simulink model "RobotX_SLAMonly"  (R2014a)
settings: Solver=FixedStepDiscrete  StartTime=0.0  StopTime=inf  FixedStep=.25  RelTol=1e-3
undefined symbols (not defined in the file): Com1, Com2, Com3, Com4, DiscIntNeverNeededParam, standard
libraries: xpcseriallib x11, simulink x3, slrtlib x3, dspmtrx3 x2, speedgoatlib x1, speedgoatlib_IO102 x1
(part 8 of 15)

== matlab function RobotX_SLAMonly/Main FSM/SLAM/Models for prediction/Model46/Dynamic Model ==
  data: F_surge input; F_sway input; Torque input; u input; surgeAccel output; v input; psi input; swayAccel output; yawAccel output
function [surgeAccel, swayAccel, yawAccel] = ...
    WAM_V_3DOF(F_surge, F_sway, Torque, u, v, psi)
%Written by Anderson Lebbad on August 12, 2014
%Last Edited:

%This function was heavily based off of Ariel Qu's Vel3DOF_IvanV1. It was
%rewritten for real-time use.

%This function will produce the transient output surge velocity of a
%linearized model of the USV. It is assumed that the vehicle is equivalent
%to two cylinders in the water.

%%%%%DEFINED VARIABLE%%%%%%
%
%   Xext = Thrust from motors
%   Next = Moment from motor
%   m = Mass of vehicle
%   Xudot = Added mass in surge direction
%   Yvdot = Added mass in sway direction
%   Nrdot = Added mass from yaw
%   xg = offset from center of gravity
%   rho = density of seawater
%   S = wetted surface area
%   R = Reynolds number
%   Cd = Coefficient of drag
%   Cdc = Coefficient of drag for sway
%   nu = Kinematic viscosity
%   L = Length overall
%   T = draft
%   B = beam
%   SA = Surface area of cylinder experiencing sway
%   Iz = moment of inertia about Z axis
%
%%%%%%

% Force/Mometns from thrusters & control surfaces...

tau = [F_surge; F_sway; Torque];

% Calculate yaw rate
persistent lastHeading
if isempty(lastHeading)
    lastHeading = psi;
end
%Sample time
ts = .1;

r = (psi - lastHeading)/ts;

% Velocity & Angular velocity vectors
vel = [u; v; 0];
omega = [0; 0; r];

%define variables
m = 145.7;         % Total mass [kg] - reduced from 102
rho = 1025.9;   % density of seawater [kg/m^3]
L = 3.91*0.85;  % Length on the waterline [m]
B = 0.426;       % Demihull beam [m]
T = B*0.2;        % Draft of the demihull [m]
p_bar = 1.0; % sidehull separation - from centerplane vessel to centerplane demihull
Iz = 262.181;    % Mass moment of inertia about z-axis [kg*m^2]
xg = 0;         % Body-Fixed coordinate system taken to be center of gravity
yg = 0;         % Symmetrical Vessel
Cd = 1.1;       % Drag coefficient for a lateral cylinder
LCG = 1.485;        % Need to know where LCG wrt stern

% Vector location of port and starboard hulls
r_port = [-LCG; -p_bar; 0];   
r_stbd = [-LCG; p_bar; 0];

% Port and starboard hull velocities
vel_port = vel + cross(omega,r_port);
vel_stbd = vel + cross(omega,r_stbd);

u_port = vel_port(1);
u_stbd = vel_stbd(1);

% Port and starboard state vectors
state_port = vel_port + omega;
state_stbd = vel_stbd + omega;

%% Added Mass
% Estimated for each hull, then multiplied by 2 to account for both hulls
Xudot = -0.05*m;

%Using strip theory to estimate added mass coefficients
Nrdot = -(4.75/2*pi*rho*p_bar*T^4 + pi*rho*T^2*((L - LCG)^3 + LCG^3)/3);
Nvdot = - pi*rho*T^2*((L - LCG)^2 - LCG^2)/2;

Yrdot = Nvdot;
Yvdot = -rho*pi*T^2*L;

% Multiply by 2:
Xudot = 2*Xudot;
Nrdot = 2*Nrdot;
Nvdot = 2*Nvdot;
Yrdot = 2*Yrdot;
Yvdot = 2*Yvdot;

%Calculate Coefficient of Drag for Sway from 1950 SNAME approximation
Cdc= 1.1 + 0.0045*L/T - 0.1*B/T + 0.016*(B/T)^2;
SA = 2*pi/4*T*L; %projected area of pontoon for two pontoons

%% Linear Drag Terms
%Total Speed
U = sqrt(u^2+v^2);

Xu = 0;
Yv = -0.5*rho*abs(v)*2*Cdc*SA; %20 was the last working number %from SNAME 1950, x2 for two cylinders
%Nr = -0.5*pi*rho*U*T^2*L^2;
Nr = -pi*rho*U*T^2*L^2*.065;
Nv = -pi*rho*U*T^2*L*.01;
Yr = pi*rho*U*T^2*L*0.2;  %from Newman approximation in Lewandowski

%% Nonlinear Drag Terms

% Drag and Moment due to drag on entire vessel - includes nonlinear and
% linear drag terms
D_port = 0.5*(0.44*u_port^3 - 0.01*u_port^2 + 19*u_port);     % Can assume that this equation also takes into account Xu - so set Xu=0
D_stbd = 0.5*(0.44*u_stbd^3 - 0.01*u_stbd^2 + 19*u_stbd);     % Can assume that this equation also takes into account Xu - so set Xu=0

tau_drag = [-(D_port + D_stbd); 0; (D_stbd - D_port)*p_bar];

Xuu = 0;

%% Maneuvering Coefficient Matrices
% Added Mass Matrix
M = [(m - Xudot)      0              0;...
    0               (m - Yvdot)     (m*xg - Yrdot);...
    0               (m*xg - Nvdot)  (Iz - Nrdot)];

%Centripetal and Added Mass Centripetal force matrices
% C_RB = [
%     0                  0                0
%     0                  0                0
%     0                  0                0
%     ];

% C_RB = [
%     0                  0                -m*(xg*r + v)
%     0                  0                -m*(yg*r - u)
%     m*(xg*r + v)       m*(yg*r - u)     0
%     ];

% C_A = -[ %negative originally
%     0                               0           0
%     0                               0           0
%     0                               0           0
%     ];

% Negating centripetal acceleration for test
C_RB = 0;
C_A = 0;

D = -[Xu  0   0;...
      0   Yv  Yr;...
      0   Nv  Nr];

% Nonlinear Drag Coefficients
D_N = -[Xuu*u   0                       0;...
        0       0                       0;...
        0       0                       0];
    
%% Calculate the port and starboard force vectors
tau_port = -(C_RB + C_A + D + D_N)*state_port;
tau_stbd = -(C_RB + C_A + D + D_N)*state_stbd;


%% Sum the force vectors
tau_tot = tau + tau_drag + tau_port + tau_stbd...
    + cross(r_port,[tau_port(1);tau_port(2);0]) + ...
    cross(r_stbd,[tau_stbd(1);tau_stbd(2);0]);

% Calculate the time derivative of the state vector

accel = M\tau_tot;

%% Separate output

surgeAccel = accel(1);
swayAccel = accel(2);
yawAccel = accel(3);

end

== matlab function RobotX_SLAMonly/Main FSM/SLAM/Models for prediction/Model48/Port Thruster Model ==
  data: portMP input; F_surge output; portAzimuth input; F_sway output; Torque output
function [F_surge,F_sway,Torque]  = PortThruster(portMP,portAzimuth)
%Approximation for Starboard Force and Moment with the input motor power
%and azimuth angle of thruster

%Longitudinal distance from center of mass
longDist =1.007;           %m

%Axial distance from center of mass
axialDist=1.485;            %m

%% Piece-wise thrust calculation

if portMP <= -51.0119
    F = .9140*portMP + 40;
elseif portMP >= 26.8367
    F = 1.658*portMP - 41.01;
else
    F = .12987*portMP;
end

%% Force components
F_surge=F*cos(portAzimuth*pi/180);       %N
F_sway=F*sin(portAzimuth*pi/180);       %N

%% Torque calculation

Torque = F_surge*longDist - F_sway*axialDist;   %N.m

end

== matlab function RobotX_SLAMonly/Main FSM/SLAM/Models for prediction/Model48/Stbd Thruster Model ==
  data: stbdMP input; F_surge output; stbdAzimuth input; F_sway output; Torque output
function [F_surge,F_sway,Torque]  = StarBoardThruster(stbdMP,stbdAzimuth)
%Approximation for Starboard Force and Moment with the input motor power
%and azimuth angle of thruster

%Longitudinal distance from center of mass
longDist =1.007;           %m

%Axial distance from center of mass
axialDist=1.485;            %m

%% Piece-wise thrust calculation

if stbdMP <= -51.0119
    F = .9140*stbdMP + 40;
elseif stbdMP >= 26.8367
    F = 1.658*stbdMP - 41.01;
else
    F = .12987*stbdMP;
end

%% Force components
F_surge=F*cos(stbdAzimuth*pi/180);       %N
F_sway=F*sin(stbdAzimuth*pi/180);       %N

%% Torque calculation

Torque = -F_surge*longDist - F_sway*axialDist;   %N.m

end

== matlab function RobotX_SLAMonly/Main FSM/SLAM/Models for prediction/Model49/Non-Holonomic Constraint ==
  data: time input; surgeAccel input; NEyaw output; swayAccel input; YawAccel input; u input; v input; gyrz input; psi input; X input; Y input
function NEyaw  = nonHolonomicNE(time,surgeAccel,swayAccel,YawAccel,u,v,gyrz,psi,X,Y)
%Written by Anderson Lebbad on August 12, 2014
%Last Edited:

%This function estimates the velocities for a new pose based off the 
%velocities and heading calculated from the dynamic model, and the current 
%pose. Uses a non-holonomic constraint for estimation.

%% Find time elapsed for integration

ts = .1;
persistent uPrev vPrev gyrzPrev psiPrev xPrev yPrev

%Initialize
if isempty(uPrev)
    uPrev = [u time];
    vPrev = [v time];
    gyrzPrev = [gyrz time];
    psiPrev = [psi time];
    xPrev = [X time];
    yPrev = [Y time];
end
    
%Update if change
if uPrev(1) ~= u
    uPrev = [u time];
end
if vPrev(1) ~= v
    vPrev = [v time];
end
if gyrzPrev(1) ~= gyrz
    gyrzPrev = [gyrz time];
end
if psiPrev(1) ~= psi
    psiPrev = [psi time];
end
if xPrev(1) ~= X
    xPrev = [X time];
end
if yPrev(1) ~= Y
    yPrev = [Y time];
end

%evaluate elapsed
uTime = ts + time - uPrev(2);
vTime = ts + time - vPrev(2);
gyrzTime = ts + time - gyrzPrev(2);
psiTime = ts + time - psiPrev(2);
xTime = ts + time - xPrev(2);
yTime = ts + time - yPrev(2);

%% Integrate inputs
surgeVel = u + surgeAccel*uTime/2;
swayVel = v + swayAccel*vTime/2;
yawVel = gyrz + YawAccel*gyrzTime/2;
yaw = psi + yawVel*psiTime/2;


%% Apply Non-holonomic constraint for NE velocities
Xd = surgeVel*cos(yaw*pi/180) - swayVel*sin(yaw*pi/180);
Yd = surgeVel*sin(yaw*pi/180) + swayVel*cos(yaw*pi/180);

%% Integrate to output NE coordinates
N = X + Xd*xTime/2;
E = Y + Yd*yTime/2;

NEyaw = [N;E;yaw];

end

== matlab function RobotX_SLAMonly/Main FSM/SLAM/Models for prediction/Model49/move_part ==
  data: PtThrust input; portMP output; PtAzimuth input; StThrust input; StAzimuth input; noiseLevel input; portAzimuth output; stbdMP output; stbdAzimuth output
function [portMP,portAzimuth,stbdMP,stbdAzimuth] = addNoise(PtThrust,...
    PtAzimuth,StThrust,StAzimuth,noiseLevel)
%Written By Anderson Lebbad on September 16, 2014
%Last Edited By:

%This function adds gaussian noise to the inputs for a particular particles
%model

portMP = normrnd(PtThrust, noiseLevel);
portAzimuth = normrnd(PtAzimuth, noiseLevel);
stbdMP = normrnd(StThrust, noiseLevel);
stbdAzimuth = normrnd(StAzimuth, noiseLevel);

end

== matlab function RobotX_SLAMonly/Main FSM/SLAM/Models for prediction/Model50/Dynamic Model ==
  data: F_surge input; F_sway input; Torque input; u input; surgeAccel output; v input; psi input; swayAccel output; yawAccel output
function [surgeAccel, swayAccel, yawAccel] = ...
    WAM_V_3DOF(F_surge, F_sway, Torque, u, v, psi)
%Written by Anderson Lebbad on August 12, 2014
%Last Edited:

%This function was heavily based off of Ariel Qu's Vel3DOF_IvanV1. It was
%rewritten for real-time use.

%This function will produce the transient output surge velocity of a
%linearized model of the USV. It is assumed that the vehicle is equivalent
%to two cylinders in the water.

%%%%%DEFINED VARIABLE%%%%%%
%
%   Xext = Thrust from motors
%   Next = Moment from motor
%   m = Mass of vehicle
%   Xudot = Added mass in surge direction
%   Yvdot = Added mass in sway direction
%   Nrdot = Added mass from yaw
%   xg = offset from center of gravity
%   rho = density of seawater
%   S = wetted surface area
%   R = Reynolds number
%   Cd = Coefficient of drag
%   Cdc = Coefficient of drag for sway
%   nu = Kinematic viscosity
%   L = Length overall
%   T = draft
%   B = beam
%   SA = Surface area of cylinder experiencing sway
%   Iz = moment of inertia about Z axis
%
%%%%%%

% Force/Mometns from thrusters & control surfaces...

tau = [F_surge; F_sway; Torque];

% Calculate yaw rate
persistent lastHeading
if isempty(lastHeading)
    lastHeading = psi;
end
%Sample time
ts = .1;

r = (psi - lastHeading)/ts;

% Velocity & Angular velocity vectors
vel = [u; v; 0];
omega = [0; 0; r];

%define variables
m = 145.7;         % Total mass [kg] - reduced from 102
rho = 1025.9;   % density of seawater [kg/m^3]
L = 3.91*0.85;  % Length on the waterline [m]
B = 0.426;       % Demihull beam [m]
T = B*0.2;        % Draft of the demihull [m]
p_bar = 1.0; % sidehull separation - from centerplane vessel to centerplane demihull
Iz = 262.181;    % Mass moment of inertia about z-axis [kg*m^2]
xg = 0;         % Body-Fixed coordinate system taken to be center of gravity
yg = 0;         % Symmetrical Vessel
Cd = 1.1;       % Drag coefficient for a lateral cylinder
LCG = 1.485;        % Need to know where LCG wrt stern

% Vector location of port and starboard hulls
r_port = [-LCG; -p_bar; 0];   
r_stbd = [-LCG; p_bar; 0];

% Port and starboard hull velocities
vel_port = vel + cross(omega,r_port);
vel_stbd = vel + cross(omega,r_stbd);

u_port = vel_port(1);
u_stbd = vel_stbd(1);

% Port and starboard state vectors
state_port = vel_port + omega;
state_stbd = vel_stbd + omega;

%% Added Mass
% Estimated for each hull, then multiplied by 2 to account for both hulls
Xudot = -0.05*m;

%Using strip theory to estimate added mass coefficients
Nrdot = -(4.75/2*pi*rho*p_bar*T^4 + pi*rho*T^2*((L - LCG)^3 + LCG^3)/3);
Nvdot = - pi*rho*T^2*((L - LCG)^2 - LCG^2)/2;

Yrdot = Nvdot;
Yvdot = -rho*pi*T^2*L;

% Multiply by 2:
Xudot = 2*Xudot;
Nrdot = 2*Nrdot;
Nvdot = 2*Nvdot;
Yrdot = 2*Yrdot;
Yvdot = 2*Yvdot;

%Calculate Coefficient of Drag for Sway from 1950 SNAME approximation
Cdc= 1.1 + 0.0045*L/T - 0.1*B/T + 0.016*(B/T)^2;
SA = 2*pi/4*T*L; %projected area of pontoon for two pontoons

%% Linear Drag Terms
%Total Speed
U = sqrt(u^2+v^2);

Xu = 0;
Yv = -0.5*rho*abs(v)*2*Cdc*SA; %20 was the last working number %from SNAME 1950, x2 for two cylinders
%Nr = -0.5*pi*rho*U*T^2*L^2;
Nr = -pi*rho*U*T^2*L^2*.065;
Nv = -pi*rho*U*T^2*L*.01;
Yr = pi*rho*U*T^2*L*0.2;  %from Newman approximation in Lewandowski

%% Nonlinear Drag Terms

% Drag and Moment due to drag on entire vessel - includes nonlinear and
% linear drag terms
D_port = 0.5*(0.44*u_port^3 - 0.01*u_port^2 + 19*u_port);     % Can assume that this equation also takes into account Xu - so set Xu=0
D_stbd = 0.5*(0.44*u_stbd^3 - 0.01*u_stbd^2 + 19*u_stbd);     % Can assume that this equation also takes into account Xu - so set Xu=0

tau_drag = [-(D_port + D_stbd); 0; (D_stbd - D_port)*p_bar];

Xuu = 0;

%% Maneuvering Coefficient Matrices
% Added Mass Matrix
M = [(m - Xudot)      0              0;...
    0               (m - Yvdot)     (m*xg - Yrdot);...
    0               (m*xg - Nvdot)  (Iz - Nrdot)];

%Centripetal and Added Mass Centripetal force matrices
% C_RB = [
%     0                  0                0
%     0                  0                0
%     0                  0                0
%     ];

% C_RB = [
%     0                  0                -m*(xg*r + v)
%     0                  0                -m*(yg*r - u)
%     m*(xg*r + v)       m*(yg*r - u)     0
%     ];

% C_A = -[ %negative originally
%     0                               0           0
%     0                               0           0
%     0                               0           0
%     ];

% Negating centripetal acceleration for test
C_RB = 0;
C_A = 0;

D = -[Xu  0   0;...
      0   Yv  Yr;...
      0   Nv  Nr];

% Nonlinear Drag Coefficients
D_N = -[Xuu*u   0                       0;...
        0       0                       0;...
        0       0                       0];
    
%% Calculate the port and starboard force vectors
tau_port = -(C_RB + C_A + D + D_N)*state_port;
tau_stbd = -(C_RB + C_A + D + D_N)*state_stbd;


%% Sum the force vectors
tau_tot = tau + tau_drag + tau_port + tau_stbd...
    + cross(r_port,[tau_port(1);tau_port(2);0]) + ...
    cross(r_stbd,[tau_stbd(1);tau_stbd(2);0]);

% Calculate the time derivative of the state vector

accel = M\tau_tot;

%% Separate output

surgeAccel = accel(1);
swayAccel = accel(2);
yawAccel = accel(3);

end

== system RobotX_SLAMonly/Main FSM/SLAM/Models for prediction/Model3 ==
  X : Inport
  Y : Inport  Port=2
  Psi : Inport  Port=3
  Nav Messages : Inport  Port=4
  Bus Selector : BusSelector  OutputSignals=Velocity.u,Velocity.v,Velocity.r,Port.PtThrust,Port.PtAzimuth,Stbd.StThrust,Stbd.StAzimuth
  Data Store Read : DataStoreRead  DataStoreName=noiseLevel
  Demux : Demux  Outputs=3
  Discrete-Time Integrator1 : DiscreteIntegrator  SampleTime=-1  ICPrevOutput=DiscIntNeverNeededParam  ICPrevScaledInput=DiscIntNeverNeededParam
  Dynamic Model : MATLAB Function  TreatAsAtomicUnit=on
  Mux : Mux  Inputs=3
  Mux1 : Mux  Inputs=3
  Non-Holonomic Constraint : MATLAB Function  TreatAsAtomicUnit=on
  Port Thruster Model : MATLAB Function  TreatAsAtomicUnit=on
  Stbd Thruster Model : MATLAB Function  TreatAsAtomicUnit=on
  Sum : Sum  Inputs=|++|
  enabled : Constant
  move_part : MATLAB Function  TreatAsAtomicUnit=on
  NEyaw : Outport
  wires:
  Sum/1 -> Demux/1  "Forces"
  Bus Selector/2 -> Non-Holonomic Constraint/6(v), Dynamic Model/5(v)  "<v>"
  Bus Selector/1 -> Non-Holonomic Constraint/5(u), Dynamic Model/4(u)  "<u>"
  Psi/1 -> Non-Holonomic Constraint/8(psi), Dynamic Model/6(psi)
  Demux/2 -> Dynamic Model/2(F_sway)
  Demux/3 -> Dynamic Model/3(Torque)
  Demux/1 -> Dynamic Model/1(F_surge)
  Mux/1 -> Sum/2
  Stbd Thruster Model/1(F_surge) -> Mux/1
  Stbd Thruster Model/3(Torque) -> Mux/3
  Stbd Thruster Model/2(F_sway) -> Mux/2
  Mux1/1 -> Sum/1
  Port Thruster Model/2(F_sway) -> Mux1/2
  Port Thruster Model/1(F_surge) -> Mux1/1
  Port Thruster Model/3(Torque) -> Mux1/3
  Dynamic Model/1(surgeAccel) -> Non-Holonomic Constraint/2(surgeAccel)
  Dynamic Model/2(swayAccel) -> Non-Holonomic Constraint/3(swayAccel)
  Dynamic Model/3(yawAccel) -> Non-Holonomic Constraint/4(YawAccel)
  Y/1 -> Non-Holonomic Constraint/10(Y)
  X/1 -> Non-Holonomic Constraint/9(X)
  Bus Selector/3 -> Non-Holonomic Constraint/7(gyrz)  "<r>"
  Non-Holonomic Constraint/1(NEyaw) -> NEyaw/1
  enabled/1 -> Discrete-Time Integrator1/1
  Discrete-Time Integrator1/1 -> Non-Holonomic Constraint/1(time)
  Nav Messages/1 -> Bus Selector/1
  Bus Selector/4 -> move_part/1(PtThrust)  "<PtThrust>"
  Bus Selector/5 -> move_part/2(PtAzimuth)  "<PtAzimuth>"
  Bus Selector/7 -> move_part/4(StAzimuth)  "<StAzimuth>"
  Bus Selector/6 -> move_part/3(StThrust)  "<StThrust>"
  move_part/1(portMP) -> Port Thruster Model/1(portMP)
  move_part/2(portAzimuth) -> Port Thruster Model/2(portAzimuth)
  move_part/3(stbdMP) -> Stbd Thruster Model/1(stbdMP)
  move_part/4(stbdAzimuth) -> Stbd Thruster Model/2(stbdAzimuth)
  Data Store Read/1 -> move_part/5(noiseLevel)

== system RobotX_SLAMonly/Main FSM/SLAM/Models for prediction/Model30 ==
  X : Inport
  Y : Inport  Port=2
  Psi : Inport  Port=3
  Nav Messages : Inport  Port=4
  Bus Selector : BusSelector  OutputSignals=Velocity.u,Velocity.v,Velocity.r,Port.PtThrust,Port.PtAzimuth,Stbd.StThrust,Stbd.StAzimuth
  Data Store Read : DataStoreRead  DataStoreName=noiseLevel
  Demux : Demux  Outputs=3
  Discrete-Time Integrator1 : DiscreteIntegrator  SampleTime=-1  ICPrevOutput=DiscIntNeverNeededParam  ICPrevScaledInput=DiscIntNeverNeededParam
  Dynamic Model : MATLAB Function  TreatAsAtomicUnit=on
  Mux : Mux  Inputs=3
  Mux1 : Mux  Inputs=3
  Non-Holonomic Constraint : MATLAB Function  TreatAsAtomicUnit=on
  Port Thruster Model : MATLAB Function  TreatAsAtomicUnit=on
  Stbd Thruster Model : MATLAB Function  TreatAsAtomicUnit=on
  Sum : Sum  Inputs=|++|
  enabled : Constant
  move_part : MATLAB Function  TreatAsAtomicUnit=on
  NEyaw : Outport
  wires:
  Sum/1 -> Demux/1  "Forces"
  Bus Selector/2 -> Non-Holonomic Constraint/6(v), Dynamic Model/5(v)  "<v>"
  Bus Selector/1 -> Non-Holonomic Constraint/5(u), Dynamic Model/4(u)  "<u>"
  Psi/1 -> Non-Holonomic Constraint/8(psi), Dynamic Model/6(psi)
  Demux/2 -> Dynamic Model/2(F_sway)
  Demux/3 -> Dynamic Model/3(Torque)
  Demux/1 -> Dynamic Model/1(F_surge)
  Mux/1 -> Sum/2
  Stbd Thruster Model/1(F_surge) -> Mux/1
  Stbd Thruster Model/3(Torque) -> Mux/3
  Stbd Thruster Model/2(F_sway) -> Mux/2
  Mux1/1 -> Sum/1
  Port Thruster Model/2(F_sway) -> Mux1/2
  Port Thruster Model/1(F_surge) -> Mux1/1
  Port Thruster Model/3(Torque) -> Mux1/3
  Dynamic Model/1(surgeAccel) -> Non-Holonomic Constraint/2(surgeAccel)
  Dynamic Model/2(swayAccel) -> Non-Holonomic Constraint/3(swayAccel)
  Dynamic Model/3(yawAccel) -> Non-Holonomic Constraint/4(YawAccel)
  Y/1 -> Non-Holonomic Constraint/10(Y)
  X/1 -> Non-Holonomic Constraint/9(X)
  Bus Selector/3 -> Non-Holonomic Constraint/7(gyrz)  "<r>"
  Non-Holonomic Constraint/1(NEyaw) -> NEyaw/1
  enabled/1 -> Discrete-Time Integrator1/1
  Discrete-Time Integrator1/1 -> Non-Holonomic Constraint/1(time)
  Nav Messages/1 -> Bus Selector/1
  Bus Selector/4 -> move_part/1(PtThrust)  "<PtThrust>"
  Bus Selector/5 -> move_part/2(PtAzimuth)  "<PtAzimuth>"
  Bus Selector/7 -> move_part/4(StAzimuth)  "<StAzimuth>"
  Bus Selector/6 -> move_part/3(StThrust)  "<StThrust>"
  move_part/1(portMP) -> Port Thruster Model/1(portMP)
  move_part/2(portAzimuth) -> Port Thruster Model/2(portAzimuth)
  move_part/3(stbdMP) -> Stbd Thruster Model/1(stbdMP)
  move_part/4(stbdAzimuth) -> Stbd Thruster Model/2(stbdAzimuth)
  Data Store Read/1 -> move_part/5(noiseLevel)

== system RobotX_SLAMonly/Main FSM/SLAM/Models for prediction/Model31 ==
  X : Inport
  Y : Inport  Port=2
  Psi : Inport  Port=3
  Nav Messages : Inport  Port=4
  Bus Selector : BusSelector  OutputSignals=Velocity.u,Velocity.v,Velocity.r,Port.PtThrust,Port.PtAzimuth,Stbd.StThrust,Stbd.StAzimuth
  Data Store Read : DataStoreRead  DataStoreName=noiseLevel
  Demux : Demux  Outputs=3
  Discrete-Time Integrator1 : DiscreteIntegrator  SampleTime=-1  ICPrevOutput=DiscIntNeverNeededParam  ICPrevScaledInput=DiscIntNeverNeededParam
  Dynamic Model : MATLAB Function  TreatAsAtomicUnit=on
  Mux : Mux  Inputs=3
  Mux1 : Mux  Inputs=3
  Non-Holonomic Constraint : MATLAB Function  TreatAsAtomicUnit=on
  Port Thruster Model : MATLAB Function  TreatAsAtomicUnit=on
  Stbd Thruster Model : MATLAB Function  TreatAsAtomicUnit=on
  Sum : Sum  Inputs=|++|
  enabled : Constant
  move_part : MATLAB Function  TreatAsAtomicUnit=on
  NEyaw : Outport
  wires:
  Sum/1 -> Demux/1  "Forces"
  Bus Selector/2 -> Non-Holonomic Constraint/6(v), Dynamic Model/5(v)  "<v>"
  Bus Selector/1 -> Non-Holonomic Constraint/5(u), Dynamic Model/4(u)  "<u>"
  Psi/1 -> Non-Holonomic Constraint/8(psi), Dynamic Model/6(psi)
  Demux/2 -> Dynamic Model/2(F_sway)
  Demux/3 -> Dynamic Model/3(Torque)
  Demux/1 -> Dynamic Model/1(F_surge)
  Mux/1 -> Sum/2
  Stbd Thruster Model/1(F_surge) -> Mux/1
  Stbd Thruster Model/3(Torque) -> Mux/3
  Stbd Thruster Model/2(F_sway) -> Mux/2
  Mux1/1 -> Sum/1
  Port Thruster Model/2(F_sway) -> Mux1/2
  Port Thruster Model/1(F_surge) -> Mux1/1
  Port Thruster Model/3(Torque) -> Mux1/3
  Dynamic Model/1(surgeAccel) -> Non-Holonomic Constraint/2(surgeAccel)
  Dynamic Model/2(swayAccel) -> Non-Holonomic Constraint/3(swayAccel)
  Dynamic Model/3(yawAccel) -> Non-Holonomic Constraint/4(YawAccel)
  Y/1 -> Non-Holonomic Constraint/10(Y)
  X/1 -> Non-Holonomic Constraint/9(X)
  Bus Selector/3 -> Non-Holonomic Constraint/7(gyrz)  "<r>"
  Non-Holonomic Constraint/1(NEyaw) -> NEyaw/1
  enabled/1 -> Discrete-Time Integrator1/1
  Discrete-Time Integrator1/1 -> Non-Holonomic Constraint/1(time)
  Nav Messages/1 -> Bus Selector/1
  Bus Selector/4 -> move_part/1(PtThrust)  "<PtThrust>"
  Bus Selector/5 -> move_part/2(PtAzimuth)  "<PtAzimuth>"
  Bus Selector/7 -> move_part/4(StAzimuth)  "<StAzimuth>"
  Bus Selector/6 -> move_part/3(StThrust)  "<StThrust>"
  move_part/1(portMP) -> Port Thruster Model/1(portMP)
  move_part/2(portAzimuth) -> Port Thruster Model/2(portAzimuth)
  move_part/3(stbdMP) -> Stbd Thruster Model/1(stbdMP)
  move_part/4(stbdAzimuth) -> Stbd Thruster Model/2(stbdAzimuth)
  Data Store Read/1 -> move_part/5(noiseLevel)

== system RobotX_SLAMonly/Main FSM/SLAM/Models for prediction/Model32 ==
  X : Inport
  Y : Inport  Port=2
  Psi : Inport  Port=3
  Nav Messages : Inport  Port=4
  Bus Selector : BusSelector  OutputSignals=Velocity.u,Velocity.v,Velocity.r,Port.PtThrust,Port.PtAzimuth,Stbd.StThrust,Stbd.StAzimuth
  Data Store Read : DataStoreRead  DataStoreName=noiseLevel
  Demux : Demux  Outputs=3
  Discrete-Time Integrator1 : DiscreteIntegrator  SampleTime=-1  ICPrevOutput=DiscIntNeverNeededParam  ICPrevScaledInput=DiscIntNeverNeededParam
  Dynamic Model : MATLAB Function  TreatAsAtomicUnit=on
  Mux : Mux  Inputs=3
  Mux1 : Mux  Inputs=3
  Non-Holonomic Constraint : MATLAB Function  TreatAsAtomicUnit=on
  Port Thruster Model : MATLAB Function  TreatAsAtomicUnit=on
  Stbd Thruster Model : MATLAB Function  TreatAsAtomicUnit=on
  Sum : Sum  Inputs=|++|
  enabled : Constant
  move_part : MATLAB Function  TreatAsAtomicUnit=on
  NEyaw : Outport
  wires:
  Sum/1 -> Demux/1  "Forces"
  Bus Selector/2 -> Non-Holonomic Constraint/6(v), Dynamic Model/5(v)  "<v>"
  Bus Selector/1 -> Non-Holonomic Constraint/5(u), Dynamic Model/4(u)  "<u>"
  Psi/1 -> Non-Holonomic Constraint/8(psi), Dynamic Model/6(psi)
  Demux/2 -> Dynamic Model/2(F_sway)
  Demux/3 -> Dynamic Model/3(Torque)
  Demux/1 -> Dynamic Model/1(F_surge)
  Mux/1 -> Sum/2
  Stbd Thruster Model/1(F_surge) -> Mux/1
  Stbd Thruster Model/3(Torque) -> Mux/3
  Stbd Thruster Model/2(F_sway) -> Mux/2
  Mux1/1 -> Sum/1
  Port Thruster Model/2(F_sway) -> Mux1/2
  Port Thruster Model/1(F_surge) -> Mux1/1
  Port Thruster Model/3(Torque) -> Mux1/3
  Dynamic Model/1(surgeAccel) -> Non-Holonomic Constraint/2(surgeAccel)
  Dynamic Model/2(swayAccel) -> Non-Holonomic Constraint/3(swayAccel)
  Dynamic Model/3(yawAccel) -> Non-Holonomic Constraint/4(YawAccel)
  Y/1 -> Non-Holonomic Constraint/10(Y)
  X/1 -> Non-Holonomic Constraint/9(X)
  Bus Selector/3 -> Non-Holonomic Constraint/7(gyrz)  "<r>"
  Non-Holonomic Constraint/1(NEyaw) -> NEyaw/1
  enabled/1 -> Discrete-Time Integrator1/1
  Discrete-Time Integrator1/1 -> Non-Holonomic Constraint/1(time)
  Nav Messages/1 -> Bus Selector/1
  Bus Selector/4 -> move_part/1(PtThrust)  "<PtThrust>"
  Bus Selector/5 -> move_part/2(PtAzimuth)  "<PtAzimuth>"
  Bus Selector/7 -> move_part/4(StAzimuth)  "<StAzimuth>"
  Bus Selector/6 -> move_part/3(StThrust)  "<StThrust>"
  move_part/1(portMP) -> Port Thruster Model/1(portMP)
  move_part/2(portAzimuth) -> Port Thruster Model/2(portAzimuth)
  move_part/3(stbdMP) -> Stbd Thruster Model/1(stbdMP)
  move_part/4(stbdAzimuth) -> Stbd Thruster Model/2(stbdAzimuth)
  Data Store Read/1 -> move_part/5(noiseLevel)

== system RobotX_SLAMonly/Main FSM/SLAM/Models for prediction/Model33 ==
  X : Inport
  Y : Inport  Port=2
  Psi : Inport  Port=3
  Nav Messages : Inport  Port=4
  Bus Selector : BusSelector  OutputSignals=Velocity.u,Velocity.v,Velocity.r,Port.PtThrust,Port.PtAzimuth,Stbd.StThrust,Stbd.StAzimuth
  Data Store Read : DataStoreRead  DataStoreName=noiseLevel
  Demux : Demux  Outputs=3
  Discrete-Time Integrator1 : DiscreteIntegrator  SampleTime=-1  ICPrevOutput=DiscIntNeverNeededParam  ICPrevScaledInput=DiscIntNeverNeededParam
  Dynamic Model : MATLAB Function  TreatAsAtomicUnit=on
  Mux : Mux  Inputs=3
  Mux1 : Mux  Inputs=3
  Non-Holonomic Constraint : MATLAB Function  TreatAsAtomicUnit=on
  Port Thruster Model : MATLAB Function  TreatAsAtomicUnit=on
  Stbd Thruster Model : MATLAB Function  TreatAsAtomicUnit=on
  Sum : Sum  Inputs=|++|
  enabled : Constant
  move_part : MATLAB Function  TreatAsAtomicUnit=on
  NEyaw : Outport
  wires:
  Sum/1 -> Demux/1  "Forces"
  Bus Selector/2 -> Non-Holonomic Constraint/6(v), Dynamic Model/5(v)  "<v>"
  Bus Selector/1 -> Non-Holonomic Constraint/5(u), Dynamic Model/4(u)  "<u>"
  Psi/1 -> Non-Holonomic Constraint/8(psi), Dynamic Model/6(psi)
  Demux/2 -> Dynamic Model/2(F_sway)
  Demux/3 -> Dynamic Model/3(Torque)
  Demux/1 -> Dynamic Model/1(F_surge)
  Mux/1 -> Sum/2
  Stbd Thruster Model/1(F_surge) -> Mux/1
  Stbd Thruster Model/3(Torque) -> Mux/3
  Stbd Thruster Model/2(F_sway) -> Mux/2
  Mux1/1 -> Sum/1
  Port Thruster Model/2(F_sway) -> Mux1/2
  Port Thruster Model/1(F_surge) -> Mux1/1
  Port Thruster Model/3(Torque) -> Mux1/3
  Dynamic Model/1(surgeAccel) -> Non-Holonomic Constraint/2(surgeAccel)
  Dynamic Model/2(swayAccel) -> Non-Holonomic Constraint/3(swayAccel)
  Dynamic Model/3(yawAccel) -> Non-Holonomic Constraint/4(YawAccel)
  Y/1 -> Non-Holonomic Constraint/10(Y)
  X/1 -> Non-Holonomic Constraint/9(X)
  Bus Selector/3 -> Non-Holonomic Constraint/7(gyrz)  "<r>"
  Non-Holonomic Constraint/1(NEyaw) -> NEyaw/1
  enabled/1 -> Discrete-Time Integrator1/1
  Discrete-Time Integrator1/1 -> Non-Holonomic Constraint/1(time)
  Nav Messages/1 -> Bus Selector/1
  Bus Selector/4 -> move_part/1(PtThrust)  "<PtThrust>"
  Bus Selector/5 -> move_part/2(PtAzimuth)  "<PtAzimuth>"
  Bus Selector/7 -> move_part/4(StAzimuth)  "<StAzimuth>"
  Bus Selector/6 -> move_part/3(StThrust)  "<StThrust>"
  move_part/1(portMP) -> Port Thruster Model/1(portMP)
  move_part/2(portAzimuth) -> Port Thruster Model/2(portAzimuth)
  move_part/3(stbdMP) -> Stbd Thruster Model/1(stbdMP)
  move_part/4(stbdAzimuth) -> Stbd Thruster Model/2(stbdAzimuth)
  Data Store Read/1 -> move_part/5(noiseLevel)

== system RobotX_SLAMonly/Main FSM/SLAM/Models for prediction/Model34 ==
  X : Inport
  Y : Inport  Port=2
  Psi : Inport  Port=3
  Nav Messages : Inport  Port=4
  Bus Selector : BusSelector  OutputSignals=Velocity.u,Velocity.v,Velocity.r,Port.PtThrust,Port.PtAzimuth,Stbd.StThrust,Stbd.StAzimuth
  Data Store Read : DataStoreRead  DataStoreName=noiseLevel
  Demux : Demux  Outputs=3
  Discrete-Time Integrator1 : DiscreteIntegrator  SampleTime=-1  ICPrevOutput=DiscIntNeverNeededParam  ICPrevScaledInput=DiscIntNeverNeededParam
  Dynamic Model : MATLAB Function  TreatAsAtomicUnit=on
  Mux : Mux  Inputs=3
  Mux1 : Mux  Inputs=3
  Non-Holonomic Constraint : MATLAB Function  TreatAsAtomicUnit=on
  Port Thruster Model : MATLAB Function  TreatAsAtomicUnit=on
  Stbd Thruster Model : MATLAB Function  TreatAsAtomicUnit=on
  Sum : Sum  Inputs=|++|
  enabled : Constant
  move_part : MATLAB Function  TreatAsAtomicUnit=on
  NEyaw : Outport
  wires:
  Sum/1 -> Demux/1  "Forces"
  Bus Selector/2 -> Non-Holonomic Constraint/6(v), Dynamic Model/5(v)  "<v>"
  Bus Selector/1 -> Non-Holonomic Constraint/5(u), Dynamic Model/4(u)  "<u>"
  Psi/1 -> Non-Holonomic Constraint/8(psi), Dynamic Model/6(psi)
  Demux/2 -> Dynamic Model/2(F_sway)
  Demux/3 -> Dynamic Model/3(Torque)
  Demux/1 -> Dynamic Model/1(F_surge)
  Mux/1 -> Sum/2
  Stbd Thruster Model/1(F_surge) -> Mux/1
  Stbd Thruster Model/3(Torque) -> Mux/3
  Stbd Thruster Model/2(F_sway) -> Mux/2
  Mux1/1 -> Sum/1
  Port Thruster Model/2(F_sway) -> Mux1/2
  Port Thruster Model/1(F_surge) -> Mux1/1
  Port Thruster Model/3(Torque) -> Mux1/3
  Dynamic Model/1(surgeAccel) -> Non-Holonomic Constraint/2(surgeAccel)
  Dynamic Model/2(swayAccel) -> Non-Holonomic Constraint/3(swayAccel)
  Dynamic Model/3(yawAccel) -> Non-Holonomic Constraint/4(YawAccel)
  Y/1 -> Non-Holonomic Constraint/10(Y)
  X/1 -> Non-Holonomic Constraint/9(X)
  Bus Selector/3 -> Non-Holonomic Constraint/7(gyrz)  "<r>"
  Non-Holonomic Constraint/1(NEyaw) -> NEyaw/1
  enabled/1 -> Discrete-Time Integrator1/1
  Discrete-Time Integrator1/1 -> Non-Holonomic Constraint/1(time)
  Nav Messages/1 -> Bus Selector/1
  Bus Selector/4 -> move_part/1(PtThrust)  "<PtThrust>"
  Bus Selector/5 -> move_part/2(PtAzimuth)  "<PtAzimuth>"
  Bus Selector/7 -> move_part/4(StAzimuth)  "<StAzimuth>"
  Bus Selector/6 -> move_part/3(StThrust)  "<StThrust>"
  move_part/1(portMP) -> Port Thruster Model/1(portMP)
  move_part/2(portAzimuth) -> Port Thruster Model/2(portAzimuth)
  move_part/3(stbdMP) -> Stbd Thruster Model/1(stbdMP)
  move_part/4(stbdAzimuth) -> Stbd Thruster Model/2(stbdAzimuth)
  Data Store Read/1 -> move_part/5(noiseLevel)

== system RobotX_SLAMonly/Main FSM/SLAM/Models for prediction/Model35 ==
  X : Inport
  Y : Inport  Port=2
  Psi : Inport  Port=3
  Nav Messages : Inport  Port=4
  Bus Selector : BusSelector  OutputSignals=Velocity.u,Velocity.v,Velocity.r,Port.PtThrust,Port.PtAzimuth,Stbd.StThrust,Stbd.StAzimuth
  Data Store Read : DataStoreRead  DataStoreName=noiseLevel
  Demux : Demux  Outputs=3
  Discrete-Time Integrator1 : DiscreteIntegrator  SampleTime=-1  ICPrevOutput=DiscIntNeverNeededParam  ICPrevScaledInput=DiscIntNeverNeededParam
  Dynamic Model : MATLAB Function  TreatAsAtomicUnit=on
  Mux : Mux  Inputs=3
  Mux1 : Mux  Inputs=3
  Non-Holonomic Constraint : MATLAB Function  TreatAsAtomicUnit=on
  Port Thruster Model : MATLAB Function  TreatAsAtomicUnit=on
  Stbd Thruster Model : MATLAB Function  TreatAsAtomicUnit=on
  Sum : Sum  Inputs=|++|
  enabled : Constant
  move_part : MATLAB Function  TreatAsAtomicUnit=on
  NEyaw : Outport
  wires:
  Sum/1 -> Demux/1  "Forces"
  Bus Selector/2 -> Non-Holonomic Constraint/6(v), Dynamic Model/5(v)  "<v>"
  Bus Selector/1 -> Non-Holonomic Constraint/5(u), Dynamic Model/4(u)  "<u>"
  Psi/1 -> Non-Holonomic Constraint/8(psi), Dynamic Model/6(psi)
  Demux/2 -> Dynamic Model/2(F_sway)
  Demux/3 -> Dynamic Model/3(Torque)
  Demux/1 -> Dynamic Model/1(F_surge)
  Mux/1 -> Sum/2
  Stbd Thruster Model/1(F_surge) -> Mux/1
  Stbd Thruster Model/3(Torque) -> Mux/3
  Stbd Thruster Model/2(F_sway) -> Mux/2
  Mux1/1 -> Sum/1
  Port Thruster Model/2(F_sway) -> Mux1/2
  Port Thruster Model/1(F_surge) -> Mux1/1
  Port Thruster Model/3(Torque) -> Mux1/3
  Dynamic Model/1(surgeAccel) -> Non-Holonomic Constraint/2(surgeAccel)
  Dynamic Model/2(swayAccel) -> Non-Holonomic Constraint/3(swayAccel)
  Dynamic Model/3(yawAccel) -> Non-Holonomic Constraint/4(YawAccel)
  Y/1 -> Non-Holonomic Constraint/10(Y)
  X/1 -> Non-Holonomic Constraint/9(X)
  Bus Selector/3 -> Non-Holonomic Constraint/7(gyrz)  "<r>"
  Non-Holonomic Constraint/1(NEyaw) -> NEyaw/1
  enabled/1 -> Discrete-Time Integrator1/1
  Discrete-Time Integrator1/1 -> Non-Holonomic Constraint/1(time)
  Nav Messages/1 -> Bus Selector/1
  Bus Selector/4 -> move_part/1(PtThrust)  "<PtThrust>"
  Bus Selector/5 -> move_part/2(PtAzimuth)  "<PtAzimuth>"
  Bus Selector/7 -> move_part/4(StAzimuth)  "<StAzimuth>"
  Bus Selector/6 -> move_part/3(StThrust)  "<StThrust>"
  move_part/1(portMP) -> Port Thruster Model/1(portMP)
  move_part/2(portAzimuth) -> Port Thruster Model/2(portAzimuth)
  move_part/3(stbdMP) -> Stbd Thruster Model/1(stbdMP)
  move_part/4(stbdAzimuth) -> Stbd Thruster Model/2(stbdAzimuth)
  Data Store Read/1 -> move_part/5(noiseLevel)

== system RobotX_SLAMonly/Main FSM/SLAM/Models for prediction/Model36 ==
  X : Inport
  Y : Inport  Port=2
  Psi : Inport  Port=3
  Nav Messages : Inport  Port=4
  Bus Selector : BusSelector  OutputSignals=Velocity.u,Velocity.v,Velocity.r,Port.PtThrust,Port.PtAzimuth,Stbd.StThrust,Stbd.StAzimuth
  Data Store Read : DataStoreRead  DataStoreName=noiseLevel
  Demux : Demux  Outputs=3
  Discrete-Time Integrator1 : DiscreteIntegrator  SampleTime=-1  ICPrevOutput=DiscIntNeverNeededParam  ICPrevScaledInput=DiscIntNeverNeededParam
  Dynamic Model : MATLAB Function  TreatAsAtomicUnit=on
  Mux : Mux  Inputs=3
  Mux1 : Mux  Inputs=3
  Non-Holonomic Constraint : MATLAB Function  TreatAsAtomicUnit=on
  Port Thruster Model : MATLAB Function  TreatAsAtomicUnit=on
  Stbd Thruster Model : MATLAB Function  TreatAsAtomicUnit=on
  Sum : Sum  Inputs=|++|
  enabled : Constant
  move_part : MATLAB Function  TreatAsAtomicUnit=on
  NEyaw : Outport
  wires:
  Sum/1 -> Demux/1  "Forces"
  Bus Selector/2 -> Non-Holonomic Constraint/6(v), Dynamic Model/5(v)  "<v>"
  Bus Selector/1 -> Non-Holonomic Constraint/5(u), Dynamic Model/4(u)  "<u>"
  Psi/1 -> Non-Holonomic Constraint/8(psi), Dynamic Model/6(psi)
  Demux/2 -> Dynamic Model/2(F_sway)
  Demux/3 -> Dynamic Model/3(Torque)
  Demux/1 -> Dynamic Model/1(F_surge)
  Mux/1 -> Sum/2
  Stbd Thruster Model/1(F_surge) -> Mux/1
  Stbd Thruster Model/3(Torque) -> Mux/3
  Stbd Thruster Model/2(F_sway) -> Mux/2
  Mux1/1 -> Sum/1
  Port Thruster Model/2(F_sway) -> Mux1/2
  Port Thruster Model/1(F_surge) -> Mux1/1
  Port Thruster Model/3(Torque) -> Mux1/3
  Dynamic Model/1(surgeAccel) -> Non-Holonomic Constraint/2(surgeAccel)
  Dynamic Model/2(swayAccel) -> Non-Holonomic Constraint/3(swayAccel)
  Dynamic Model/3(yawAccel) -> Non-Holonomic Constraint/4(YawAccel)
  Y/1 -> Non-Holonomic Constraint/10(Y)
  X/1 -> Non-Holonomic Constraint/9(X)
  Bus Selector/3 -> Non-Holonomic Constraint/7(gyrz)  "<r>"
  Non-Holonomic Constraint/1(NEyaw) -> NEyaw/1
  enabled/1 -> Discrete-Time Integrator1/1
  Discrete-Time Integrator1/1 -> Non-Holonomic Constraint/1(time)
  Nav Messages/1 -> Bus Selector/1
  Bus Selector/4 -> move_part/1(PtThrust)  "<PtThrust>"
  Bus Selector/5 -> move_part/2(PtAzimuth)  "<PtAzimuth>"
  Bus Selector/7 -> move_part/4(StAzimuth)  "<StAzimuth>"
  Bus Selector/6 -> move_part/3(StThrust)  "<StThrust>"
  move_part/1(portMP) -> Port Thruster Model/1(portMP)
  move_part/2(portAzimuth) -> Port Thruster Model/2(portAzimuth)
  move_part/3(stbdMP) -> Stbd Thruster Model/1(stbdMP)
  move_part/4(stbdAzimuth) -> Stbd Thruster Model/2(stbdAzimuth)
  Data Store Read/1 -> move_part/5(noiseLevel)

== system RobotX_SLAMonly/Main FSM/SLAM/Models for prediction/Model37 ==
  X : Inport
  Y : Inport  Port=2
  Psi : Inport  Port=3
  Nav Messages : Inport  Port=4
  Bus Selector : BusSelector  OutputSignals=Velocity.u,Velocity.v,Velocity.r,Port.PtThrust,Port.PtAzimuth,Stbd.StThrust,Stbd.StAzimuth
  Data Store Read : DataStoreRead  DataStoreName=noiseLevel
  Demux : Demux  Outputs=3
  Discrete-Time Integrator1 : DiscreteIntegrator  SampleTime=-1  ICPrevOutput=DiscIntNeverNeededParam  ICPrevScaledInput=DiscIntNeverNeededParam
  Dynamic Model : MATLAB Function  TreatAsAtomicUnit=on
  Mux : Mux  Inputs=3
  Mux1 : Mux  Inputs=3
  Non-Holonomic Constraint : MATLAB Function  TreatAsAtomicUnit=on
  Port Thruster Model : MATLAB Function  TreatAsAtomicUnit=on
  Stbd Thruster Model : MATLAB Function  TreatAsAtomicUnit=on
  Sum : Sum  Inputs=|++|
  enabled : Constant
  move_part : MATLAB Function  TreatAsAtomicUnit=on
  NEyaw : Outport
  wires:
  Sum/1 -> Demux/1  "Forces"
  Bus Selector/2 -> Non-Holonomic Constraint/6(v), Dynamic Model/5(v)  "<v>"
  Bus Selector/1 -> Non-Holonomic Constraint/5(u), Dynamic Model/4(u)  "<u>"
  Psi/1 -> Non-Holonomic Constraint/8(psi), Dynamic Model/6(psi)
  Demux/2 -> Dynamic Model/2(F_sway)
  Demux/3 -> Dynamic Model/3(Torque)
  Demux/1 -> Dynamic Model/1(F_surge)
  Mux/1 -> Sum/2
  Stbd Thruster Model/1(F_surge) -> Mux/1
  Stbd Thruster Model/3(Torque) -> Mux/3
  Stbd Thruster Model/2(F_sway) -> Mux/2
  Mux1/1 -> Sum/1
  Port Thruster Model/2(F_sway) -> Mux1/2
  Port Thruster Model/1(F_surge) -> Mux1/1
  Port Thruster Model/3(Torque) -> Mux1/3
  Dynamic Model/1(surgeAccel) -> Non-Holonomic Constraint/2(surgeAccel)
  Dynamic Model/2(swayAccel) -> Non-Holonomic Constraint/3(swayAccel)
  Dynamic Model/3(yawAccel) -> Non-Holonomic Constraint/4(YawAccel)
  Y/1 -> Non-Holonomic Constraint/10(Y)
  X/1 -> Non-Holonomic Constraint/9(X)
  Bus Selector/3 -> Non-Holonomic Constraint/7(gyrz)  "<r>"
  Non-Holonomic Constraint/1(NEyaw) -> NEyaw/1
  enabled/1 -> Discrete-Time Integrator1/1
  Discrete-Time Integrator1/1 -> Non-Holonomic Constraint/1(time)
  Nav Messages/1 -> Bus Selector/1
  Bus Selector/4 -> move_part/1(PtThrust)  "<PtThrust>"
  Bus Selector/5 -> move_part/2(PtAzimuth)  "<PtAzimuth>"
  Bus Selector/7 -> move_part/4(StAzimuth)  "<StAzimuth>"
  Bus Selector/6 -> move_part/3(StThrust)  "<StThrust>"
  move_part/1(portMP) -> Port Thruster Model/1(portMP)
  move_part/2(portAzimuth) -> Port Thruster Model/2(portAzimuth)
  move_part/3(stbdMP) -> Stbd Thruster Model/1(stbdMP)
  move_part/4(stbdAzimuth) -> Stbd Thruster Model/2(stbdAzimuth)
  Data Store Read/1 -> move_part/5(noiseLevel)

== system RobotX_SLAMonly/Main FSM/SLAM/Models for prediction/Model38 ==
  X : Inport
  Y : Inport  Port=2
  Psi : Inport  Port=3
  Nav Messages : Inport  Port=4
  Bus Selector : BusSelector  OutputSignals=Velocity.u,Velocity.v,Velocity.r,Port.PtThrust,Port.PtAzimuth,Stbd.StThrust,Stbd.StAzimuth
  Data Store Read : DataStoreRead  DataStoreName=noiseLevel
  Demux : Demux  Outputs=3
  Discrete-Time Integrator1 : DiscreteIntegrator  SampleTime=-1  ICPrevOutput=DiscIntNeverNeededParam  ICPrevScaledInput=DiscIntNeverNeededParam
  Dynamic Model : MATLAB Function  TreatAsAtomicUnit=on
  Mux : Mux  Inputs=3
  Mux1 : Mux  Inputs=3
  Non-Holonomic Constraint : MATLAB Function  TreatAsAtomicUnit=on
  Port Thruster Model : MATLAB Function  TreatAsAtomicUnit=on
  Stbd Thruster Model : MATLAB Function  TreatAsAtomicUnit=on
  Sum : Sum  Inputs=|++|
  enabled : Constant
  move_part : MATLAB Function  TreatAsAtomicUnit=on
  NEyaw : Outport
  wires:
  Sum/1 -> Demux/1  "Forces"
  Bus Selector/2 -> Non-Holonomic Constraint/6(v), Dynamic Model/5(v)  "<v>"
  Bus Selector/1 -> Non-Holonomic Constraint/5(u), Dynamic Model/4(u)  "<u>"
  Psi/1 -> Non-Holonomic Constraint/8(psi), Dynamic Model/6(psi)
  Demux/2 -> Dynamic Model/2(F_sway)
  Demux/3 -> Dynamic Model/3(Torque)
  Demux/1 -> Dynamic Model/1(F_surge)
  Mux/1 -> Sum/2
  Stbd Thruster Model/1(F_surge) -> Mux/1
  Stbd Thruster Model/3(Torque) -> Mux/3
  Stbd Thruster Model/2(F_sway) -> Mux/2
  Mux1/1 -> Sum/1
  Port Thruster Model/2(F_sway) -> Mux1/2
  Port Thruster Model/1(F_surge) -> Mux1/1
  Port Thruster Model/3(Torque) -> Mux1/3
  Dynamic Model/1(surgeAccel) -> Non-Holonomic Constraint/2(surgeAccel)
  Dynamic Model/2(swayAccel) -> Non-Holonomic Constraint/3(swayAccel)
  Dynamic Model/3(yawAccel) -> Non-Holonomic Constraint/4(YawAccel)
  Y/1 -> Non-Holonomic Constraint/10(Y)
  X/1 -> Non-Holonomic Constraint/9(X)
  Bus Selector/3 -> Non-Holonomic Constraint/7(gyrz)  "<r>"
  Non-Holonomic Constraint/1(NEyaw) -> NEyaw/1
  enabled/1 -> Discrete-Time Integrator1/1
  Discrete-Time Integrator1/1 -> Non-Holonomic Constraint/1(time)
  Nav Messages/1 -> Bus Selector/1
  Bus Selector/4 -> move_part/1(PtThrust)  "<PtThrust>"
  Bus Selector/5 -> move_part/2(PtAzimuth)  "<PtAzimuth>"
  Bus Selector/7 -> move_part/4(StAzimuth)  "<StAzimuth>"
  Bus Selector/6 -> move_part/3(StThrust)  "<StThrust>"
  move_part/1(portMP) -> Port Thruster Model/1(portMP)
  move_part/2(portAzimuth) -> Port Thruster Model/2(portAzimuth)
  move_part/3(stbdMP) -> Stbd Thruster Model/1(stbdMP)
  move_part/4(stbdAzimuth) -> Stbd Thruster Model/2(stbdAzimuth)
  Data Store Read/1 -> move_part/5(noiseLevel)

== system RobotX_SLAMonly/Main FSM/SLAM/Models for prediction/Model39 ==
  X : Inport
  Y : Inport  Port=2
  Psi : Inport  Port=3
  Nav Messages : Inport  Port=4
  Bus Selector : BusSelector  OutputSignals=Velocity.u,Velocity.v,Velocity.r,Port.PtThrust,Port.PtAzimuth,Stbd.StThrust,Stbd.StAzimuth
  Data Store Read : DataStoreRead  DataStoreName=noiseLevel
  Demux : Demux  Outputs=3
  Discrete-Time Integrator1 : DiscreteIntegrator  SampleTime=-1  ICPrevOutput=DiscIntNeverNeededParam  ICPrevScaledInput=DiscIntNeverNeededParam
  Dynamic Model : MATLAB Function  TreatAsAtomicUnit=on
  Mux : Mux  Inputs=3
  Mux1 : Mux  Inputs=3
  Non-Holonomic Constraint : MATLAB Function  TreatAsAtomicUnit=on
  Port Thruster Model : MATLAB Function  TreatAsAtomicUnit=on
  Stbd Thruster Model : MATLAB Function  TreatAsAtomicUnit=on
  Sum : Sum  Inputs=|++|
  enabled : Constant
  move_part : MATLAB Function  TreatAsAtomicUnit=on
  NEyaw : Outport
  wires:
  Sum/1 -> Demux/1  "Forces"
  Bus Selector/2 -> Non-Holonomic Constraint/6(v), Dynamic Model/5(v)  "<v>"
  Bus Selector/1 -> Non-Holonomic Constraint/5(u), Dynamic Model/4(u)  "<u>"
  Psi/1 -> Non-Holonomic Constraint/8(psi), Dynamic Model/6(psi)
  Demux/2 -> Dynamic Model/2(F_sway)
  Demux/3 -> Dynamic Model/3(Torque)
  Demux/1 -> Dynamic Model/1(F_surge)
  Mux/1 -> Sum/2
  Stbd Thruster Model/1(F_surge) -> Mux/1
  Stbd Thruster Model/3(Torque) -> Mux/3
  Stbd Thruster Model/2(F_sway) -> Mux/2
  Mux1/1 -> Sum/1
  Port Thruster Model/2(F_sway) -> Mux1/2
  Port Thruster Model/1(F_surge) -> Mux1/1
  Port Thruster Model/3(Torque) -> Mux1/3
  Dynamic Model/1(surgeAccel) -> Non-Holonomic Constraint/2(surgeAccel)
  Dynamic Model/2(swayAccel) -> Non-Holonomic Constraint/3(swayAccel)
  Dynamic Model/3(yawAccel) -> Non-Holonomic Constraint/4(YawAccel)
  Y/1 -> Non-Holonomic Constraint/10(Y)
  X/1 -> Non-Holonomic Constraint/9(X)
  Bus Selector/3 -> Non-Holonomic Constraint/7(gyrz)  "<r>"
  Non-Holonomic Constraint/1(NEyaw) -> NEyaw/1
  enabled/1 -> Discrete-Time Integrator1/1
  Discrete-Time Integrator1/1 -> Non-Holonomic Constraint/1(time)
  Nav Messages/1 -> Bus Selector/1
  Bus Selector/4 -> move_part/1(PtThrust)  "<PtThrust>"
  Bus Selector/5 -> move_part/2(PtAzimuth)  "<PtAzimuth>"
  Bus Selector/7 -> move_part/4(StAzimuth)  "<StAzimuth>"
  Bus Selector/6 -> move_part/3(StThrust)  "<StThrust>"
  move_part/1(portMP) -> Port Thruster Model/1(portMP)
  move_part/2(portAzimuth) -> Port Thruster Model/2(portAzimuth)
  move_part/3(stbdMP) -> Stbd Thruster Model/1(stbdMP)
  move_part/4(stbdAzimuth) -> Stbd Thruster Model/2(stbdAzimuth)
  Data Store Read/1 -> move_part/5(noiseLevel)

== system RobotX_SLAMonly/Main FSM/SLAM/Models for prediction/Model4 ==
  X : Inport
  Y : Inport  Port=2
  Psi : Inport  Port=3
  Nav Messages : Inport  Port=4
  Bus Selector : BusSelector  OutputSignals=Velocity.u,Velocity.v,Velocity.r,Port.PtThrust,Port.PtAzimuth,Stbd.StThrust,Stbd.StAzimuth
  Data Store Read : DataStoreRead  DataStoreName=noiseLevel
  Demux : Demux  Outputs=3
  Discrete-Time Integrator1 : DiscreteIntegrator  SampleTime=-1  ICPrevOutput=DiscIntNeverNeededParam  ICPrevScaledInput=DiscIntNeverNeededParam
  Dynamic Model : MATLAB Function  TreatAsAtomicUnit=on
  Mux : Mux  Inputs=3
  Mux1 : Mux  Inputs=3
  Non-Holonomic Constraint : MATLAB Function  TreatAsAtomicUnit=on
  Port Thruster Model : MATLAB Function  TreatAsAtomicUnit=on
  Stbd Thruster Model : MATLAB Function  TreatAsAtomicUnit=on
  Sum : Sum  Inputs=|++|
  enabled : Constant
  move_part : MATLAB Function  TreatAsAtomicUnit=on
  NEyaw : Outport
  wires:
  Sum/1 -> Demux/1  "Forces"
  Bus Selector/2 -> Non-Holonomic Constraint/6(v), Dynamic Model/5(v)  "<v>"
  Bus Selector/1 -> Non-Holonomic Constraint/5(u), Dynamic Model/4(u)  "<u>"
  Psi/1 -> Non-Holonomic Constraint/8(psi), Dynamic Model/6(psi)
  Demux/2 -> Dynamic Model/2(F_sway)
  Demux/3 -> Dynamic Model/3(Torque)
  Demux/1 -> Dynamic Model/1(F_surge)
  Mux/1 -> Sum/2
  Stbd Thruster Model/1(F_surge) -> Mux/1
  Stbd Thruster Model/3(Torque) -> Mux/3
  Stbd Thruster Model/2(F_sway) -> Mux/2
  Mux1/1 -> Sum/1
  Port Thruster Model/2(F_sway) -> Mux1/2
  Port Thruster Model/1(F_surge) -> Mux1/1
  Port Thruster Model/3(Torque) -> Mux1/3
  Dynamic Model/1(surgeAccel) -> Non-Holonomic Constraint/2(surgeAccel)
  Dynamic Model/2(swayAccel) -> Non-Holonomic Constraint/3(swayAccel)
  Dynamic Model/3(yawAccel) -> Non-Holonomic Constraint/4(YawAccel)
  Y/1 -> Non-Holonomic Constraint/10(Y)
  X/1 -> Non-Holonomic Constraint/9(X)
  Bus Selector/3 -> Non-Holonomic Constraint/7(gyrz)  "<r>"
  Non-Holonomic Constraint/1(NEyaw) -> NEyaw/1
  enabled/1 -> Discrete-Time Integrator1/1
  Discrete-Time Integrator1/1 -> Non-Holonomic Constraint/1(time)
  Nav Messages/1 -> Bus Selector/1
  Bus Selector/4 -> move_part/1(PtThrust)  "<PtThrust>"
  Bus Selector/5 -> move_part/2(PtAzimuth)  "<PtAzimuth>"
  Bus Selector/7 -> move_part/4(StAzimuth)  "<StAzimuth>"
  Bus Selector/6 -> move_part/3(StThrust)  "<StThrust>"
  move_part/1(portMP) -> Port Thruster Model/1(portMP)
  move_part/2(portAzimuth) -> Port Thruster Model/2(portAzimuth)
  move_part/3(stbdMP) -> Stbd Thruster Model/1(stbdMP)
  move_part/4(stbdAzimuth) -> Stbd Thruster Model/2(stbdAzimuth)
  Data Store Read/1 -> move_part/5(noiseLevel)
